simulink model "final_sim_with_control"  (R2024b)
settings: Solver=VariableStepAuto  StartTime=0.0  StopTime=20  RelTol=1e-4
libraries: spsDCVoltageSourceLib x2, spsSeriesRLCBranchLib x2, spsVoltageMeasurementLib x2, spsCurrentMeasurementLib x1, spsDCMachineLib x1, spsDiodeLib x1, spsMosfetLib x1, eePowerMeasurement x1, spsTriangleGeneratorLib x1, sps_lib x1
settings Model: SimulationMode=accelerator  Creator=sefer  LastModifiedBy=PC

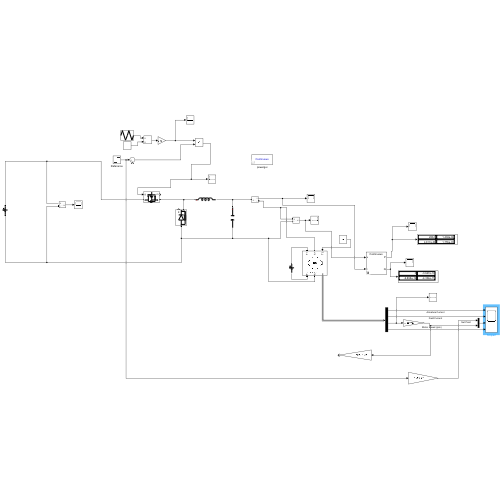
[thumbnail: Simulink's stored preview of the top-level diagram]
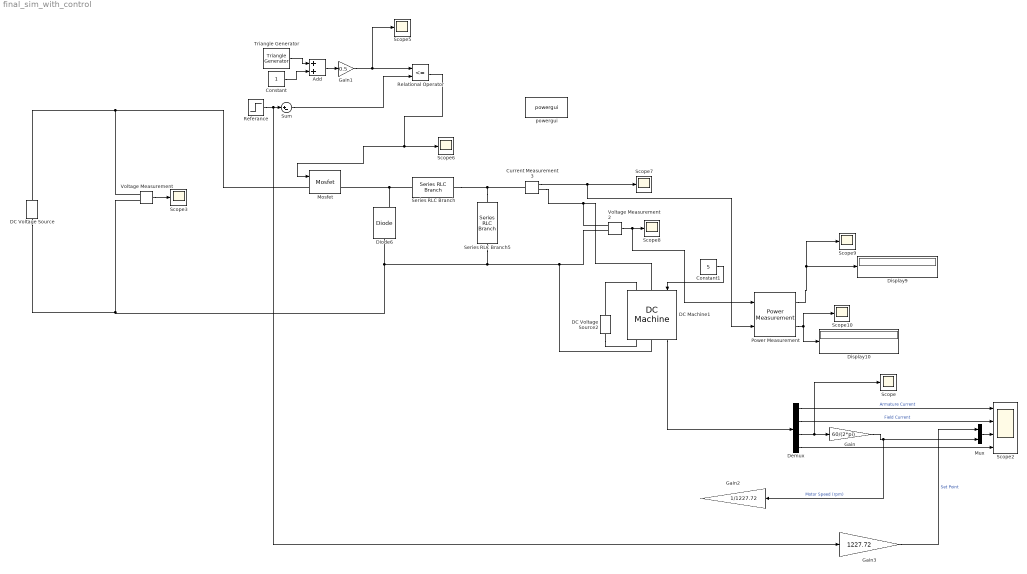
== system final_sim_with_control ==
  Add : Sum
  Constant : Constant
  Constant1 : Constant  Value=5
  Current Measurement3 : spsCurrentMeasurementLib/Current Measurement  PhasorSimulation=off  OutputType=Complex  PSBequivalent=0
  DC Machine1 : spsDCMachineLib/DC Machine  PresetModel=No  MechanicalLoad=Torque TL  FieldType=Wound  ShowDetailedParameters=on  MeasurementBus=off  RLa="[ 1.07  0.0245]"  RLf="[ 210  23]"  Laf=1.8  MachineConstant=Torque constant (N.m/A)  Ke=1.8  Kt=1.8  J=1  Bm=0  Tf=0  w0=0  Ifinit=1.04761904761905  TsPowergui=0  TsBlock=-1
  DC Voltage Source : spsDCVoltageSourceLib/DC Voltage Source  Amplitude=540  Measurements=None
  DC Voltage Source2 : spsDCVoltageSourceLib/DC Voltage Source  Amplitude=220  Measurements=None
  Demux : Demux
  Diode6 : spsDiodeLib/Diode  Ron=0.001  Lon=0  Vf=0.8  IC=0  UseSnubber=0  Rs=500  Cs=250e-9  Measurements=on
  Display10 : Display
  Display9 : Display
  Gain : Gain  Gain=60/(2*pi)
  Gain1 : Gain  Gain=0.5
  Gain2 : Gain  Gain=1/1227.72
  Gain3 : Gain  Gain=1227.72
  Mosfet : spsMosfetLib/Mosfet  Ron=0.1  Lon=0  Rd=0.01  Vfd=0  IC=0  Rs=1e5  Cs=inf  Measurements=on
  Mux : Mux  Inputs=2
  Power Measurement : eePowerMeasurement/Power Measurement  LabelModeActiveChoice=Continuous  F=60  K=[0 1 2 3]  Ts=0
  Referance : Step  Time=3  SampleTime=0
  Relational Operator : RelationalOperator  Operator=<=  OutDataTypeStr=boolean  RndMeth=Simplest  InputSameDT=off
  Scope{,3,5..10} (8 alike) : Scope
  Scope2 : Scope  NumInputPorts=4
  Series RLC Branch : spsSeriesRLCBranchLib/Series RLC Branch  LConnTagsString=__new0  RConnTagsString=__new0  BranchType=L  Resistance=1  Inductance=10e-3  SetiL0=off  InitialCurrent=0  Capacitance=1e-6  Setx0=off  InitialVoltage=0  Measurements=None
  Series RLC Branch5 : spsSeriesRLCBranchLib/Series RLC Branch  LConnTagsString=__new0  RConnTagsString=__new0  BranchType=C  Resistance=1  Inductance=1e-3  SetiL0=off  InitialCurrent=0  Capacitance=100e-6  Setx0=off  InitialVoltage=0  Measurements=None
  Sum : Sum  Inputs=|+-
  Triangle Generator : spsTriangleGeneratorLib/Triangle Generator  Freq=1e3  Phase=90  Ts=0
  Voltage Measurement : spsVoltageMeasurementLib/Voltage Measurement  PhasorSimulation=off  OutputType=Complex  PSBequivalent=0
  Voltage Measurement2 : spsVoltageMeasurementLib/Voltage Measurement  PhasorSimulation=off  OutputType=Complex  PSBequivalent=0
  powergui : sps_lib/powergui  Priority=1  SimulationMode=Continuous  SampleTime=50e-6  frequency=60  Iterations=50  frequencyindice=0  Pbase=100e6  ErrMax=1e-4  UnitsV=kV  UnitsW=MW  buscounter=0  FunctionMessages=off  echomessages=off  EnableUseOfTLC=off  CurrentSourceSwitches=off  DisableSnubberDevices=off  DisableRonSwitches=off  DisableVfSwitches=off  DisplayEquations=off  AutomaticDiscreteSolvers=off  SolverType=Tustin/Backward Euler (TBE)  Interpol=off  ExternalGateDelay=off  methode=off  Ts=100  x0status=blocks  SPID=on  SwTol=0  HookPort=off  NonlinearTolerance=1e-4  nMaxIteration=100  ContinueOnMaxIteration=off  RestoreLinks=warning  ResistiveCurrentMeasurement=off  Frange=[0:2:500]  Ylog=off  Xlog=on  ShowGrid=off  save=off  variable=ZData  structure=0  ZoomFFT=off  StartTime=0.0  cycles=1  DisplayStyle=1  fundamental=60  FreqAxis=off  MaxFrequency=1000  frequencyindicesteady=1  RmsSteady=1  display=off
  wires:
  Voltage Measurement/1 -> Scope3/1
  Voltage Measurement2/1 -> Power Measurement/1, Scope8/1
  Current Measurement3/1 -> Power Measurement/2, Scope7/1
  DC Machine1/1 -> Demux/1
  Gain/1 -> Gain2/1, Mux/2  "Motor Speed (rpm)"
  Demux/1 -> Scope2/1  "Armature Current"
  Demux/2 -> Scope2/2  "Field Current"
  Demux/4 -> Scope2/4
  Mux/1 -> Scope2/3
  Demux/3 -> Scope/1, Gain/1
  Relational Operator/1 -> Mosfet/1, Scope6/1
  Power Measurement/2 -> Scope10/1, Display10/1
  Power Measurement/1 -> Scope9/1, Display9/1
  Constant/1 -> Add/2
  Triangle Generator/1 -> Add/1
  Add/1 -> Gain1/1
  Gain1/1 -> Scope5/1, Relational Operator/1
  Referance/1 -> Gain3/1, Sum/1
  Sum/1 -> Relational Operator/2
  Gain3/1 -> Mux/1  "Set Point"
  Constant1/1 -> DC Machine1/1
  connections:
  Series RLC Branch5/RConn1 -- DC Machine1/RConn1 -- Voltage Measurement2/LConn2 -- DC Voltage Source/LConn1 -- Voltage Measurement/LConn2 -- Diode6/LConn1
  Voltage Measurement/LConn1 -- DC Voltage Source/RConn1 -- Mosfet/LConn1
  Series RLC Branch/LConn1 -- Mosfet/RConn1 -- Diode6/RConn1
  Series RLC Branch5/LConn1 -- Series RLC Branch/RConn1 -- Current Measurement3/LConn1
  Voltage Measurement2/LConn1 -- Current Measurement3/RConn1 -- DC Machine1/LConn1
  DC Voltage Source2/RConn1 -- DC Machine1/LConn2
  DC Voltage Source2/LConn1 -- DC Machine1/RConn2
